simulink model "IIR1"  (Simulink 8.1)
settings: Solver=ode45  StartTime=0.0  StopTime=simtime  RelTol=1e-3
values from neighbouring files (symbols this model uses):
  K2 = 0.132813    [cic_test.m]    (also in lf_param.m = 0.0253754; lf_test.m = 0.1328)
  K3 = 0.90625    [cic_test.m]    (also in lf_param.m = 0.850128; lf_test.m)
  R = 8    [cic_test.m]    (also in lf_test.m)
  ts_in = 1/625/1e6    (= 1.6e-09)    [cic_test.m]    (also in lf_test.m)
settings Model: MinMaxOverflowLogging=MinMaxAndOverflow  Creator=amr  LastModifiedBy=amr
settings DataIOCC: SignalLoggingSaveFormat=Dataset
settings OptimizationCC: ExpressionDepthLimit=128
settings DebuggingCC: FcnCallInpInsideContextMsg=EnableAllAsError  LoggingUnavailableSignals=none
settings GRTTargetCC: CombineOutputUpdateFcns=on  GRTInterface=off

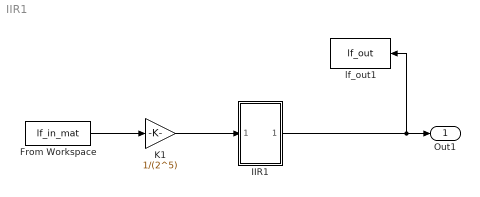
== system IIR1 ==
  From Workspace : FromWorkspace  VariableName=lf_in_mat  OutDataTypeStr=double  SampleTime=ts_in*R  Interpolate=off  OutputAfterFinalValue=Holding final value
  IIR1 : Subsystem
  K1 : Gain  Gain=1/(2^5)  ParamDataTypeStr=double  OutDataTypeStr=double  SaturateOnIntegerOverflow=on
  lf_out1 : ToWorkspace  VariableName=lf_out  SampleTime=-1
  Out1 : Outport
  wires:
  From Workspace/1 -> K1/1
  K1/1 -> IIR1/1(In1)
  IIR1/1(Out1) -> lf_out1/1, Out1/1

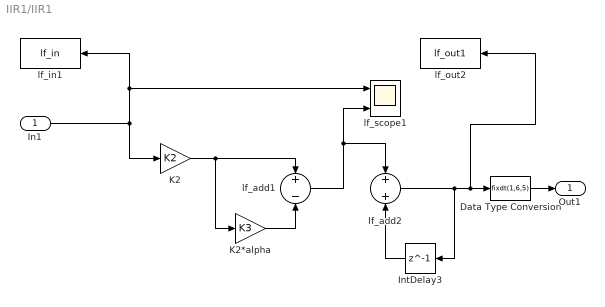
== system IIR1/IIR1 ==
  In1 : Inport
  Data Type Conversion : DataTypeConversion  OutDataTypeStr=fixdt(1,6,5)
  IntDelay3 : Delay  DelayLength=1  InitialCondition=0
  K2 : Gain  Gain=K2  ParamDataTypeStr=fixdt(1,6,7)  OutDataTypeStr=fixdt(1,7,8)  SaturateOnIntegerOverflow=on
  K2*alpha : Gain  Gain=K3  ParamDataTypeStr=fixdt(1,6,5)  OutDataTypeStr=fixdt(1,8,9)  SaturateOnIntegerOverflow=on
  lf_add1 : Sum  Inputs=+-  AccumDataTypeStr=double  OutDataTypeStr=double
  lf_add2 : Sum  AccumDataTypeStr=double  OutDataTypeStr=fixdt(1,10,9)  SaturateOnIntegerOverflow=on
  lf_in1 : ToWorkspace  VariableName=lf_in  SampleTime=-1
  lf_out2 : ToWorkspace  VariableName=lf_out1  SampleTime=-1
  lf_scope1 : Scope  NumInputPorts=2
      settings: TimeRange=1.8e-06  YMin=0~-5  YMax=20~5
  Out1 : Outport
  wires:
  lf_add2/1 -> IntDelay3/1, Data Type Conversion/1, lf_out2/1
  lf_add1/1 -> lf_add2/1, lf_scope1/2
  K2*alpha/1 -> lf_add1/2
  IntDelay3/1 -> lf_add2/2
  K2/1 -> lf_add1/1, K2*alpha/1
  In1/1 -> K2/1, lf_in1/1, lf_scope1/1
  Data Type Conversion/1 -> Out1/1
